simulink model "Spiralmovement"  (Simulink 7.1)
settings: Solver=ode45  StartTime=0.0  StopTime=10.0  MaxStep=0.01  RelTol=1e-3
settings Model: Creator=Meisel  LastModifiedBy=Meisel

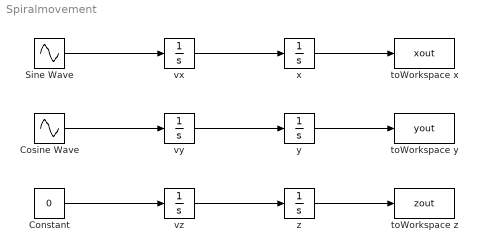
== system Spiralmovement ==
  Constant : Constant  Value=0  OutDataType=sfix(16)  OutScaling=2^0
  Cosine Wave : Sin  Amplitude=-pi*pi  Frequency=pi  Phase=pi/2  SampleTime=0
  Sine Wave : Sin  Amplitude=-pi*pi  Frequency=pi  SampleTime=0
  toWorkspace x : ToWorkspace  VariableName=xout  SampleTime=-1  SaveFormat=Array
  toWorkspace y : ToWorkspace  VariableName=yout  SampleTime=-1  SaveFormat=Array
  toWorkspace z : ToWorkspace  VariableName=zout  SampleTime=-1  SaveFormat=Array
  vx : Integrator  InitialCondition=pi
  vy : Integrator
  vz : Integrator  InitialCondition=1
  x : Integrator
  y : Integrator  InitialCondition=1
  z : Integrator
  wires:
  vx/1 -> x/1
  Sine Wave/1 -> vx/1
  x/1 -> toWorkspace x/1
  vy/1 -> y/1
  Cosine Wave/1 -> vy/1
  y/1 -> toWorkspace y/1
  vz/1 -> z/1
  Constant/1 -> vz/1
  z/1 -> toWorkspace z/1
